simulink model "Farmakokinetika"  (R2022b)
settings: Solver=VariableStepAuto  StartTime=0.0  StopTime=600  RelTol=1e-3
values from neighbouring files (symbols this model uses):
  Gb = 153    [params.m]
  Ib = 6.5    [params.m]
  ki = Pop(i,3)    [fitness.m]    (also in gen3.m = best_ch(3,end); params.m = 0.1629)
  p2 = Pop(i,1)    [fitness_dk.m]    (also in params.m = best_ch(1,end))
  Sg = 0    [params.m]
  Si = Pop(i,2)    [fitness_dk.m]    (also in params.m = best_ch(2,end))
  Ti = Pop(i,1)    [fitness.m]    (also in gen3.m = best_ch(1,end); params.m = 45.383)
  v = 281.218    [fitness.m]    (also in fitness_dk.m; gen3.m = 281.28; params.m = 281.28)
  Vg = 1.467    [params.m]
  Vi = Pop(i,2)    [fitness.m]    (also in gen3.m = best_ch(2,end); params.m = 139.094)
  weight = 64.4    [params.m]
settings Model: Creator=DFUNDO  LastModifiedBy=DFUNDO

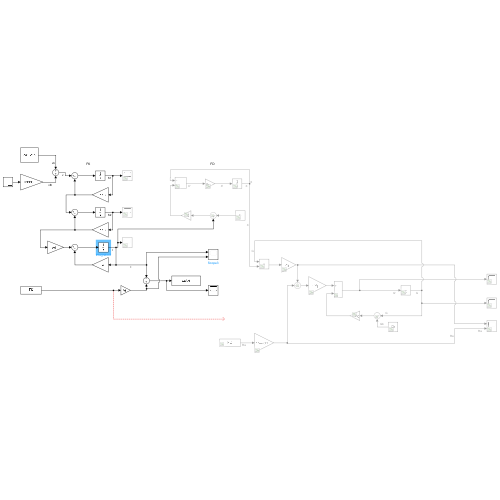
[thumbnail: Simulink's stored preview of the top-level diagram]
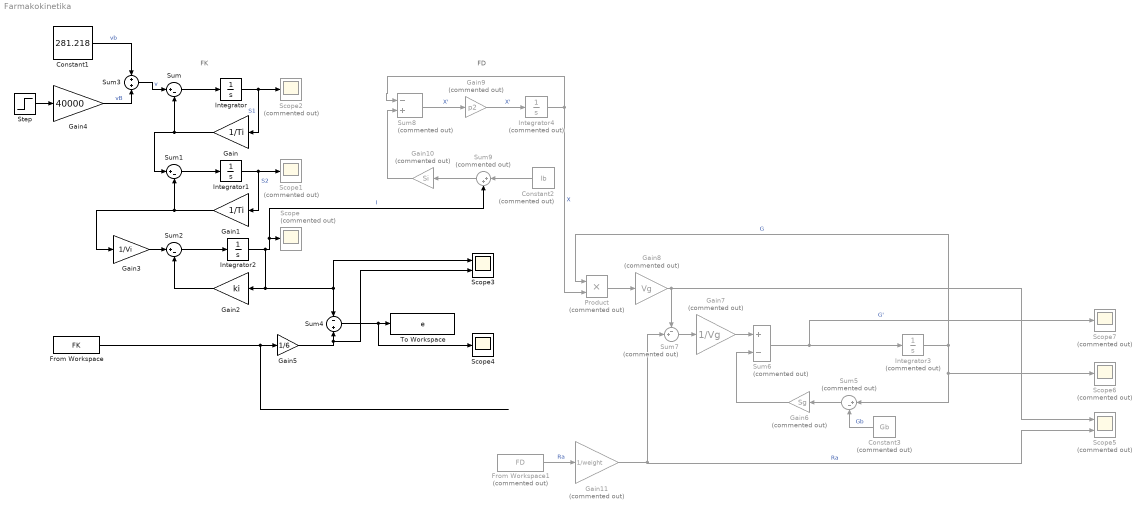
== system Farmakokinetika ==
  note: FD
  note: FK
  Constant1 : Constant  Value=281.218
  Constant2 : Constant  Commented=on  Value=Ib
  Constant3 : Constant  Commented=on  Value=Gb
  From Workspace : FromWorkspace  VariableName=FK
  From Workspace1 : FromWorkspace  Commented=on  VariableName=FD
  Gain : Gain  Gain=1/Ti
  Gain1 : Gain  Gain=1/Ti
  Gain10 : Gain  Commented=on  Gain=Si
  Gain11 : Gain  Commented=on  Gain=1/weight
  Gain2 : Gain  Gain=ki
  Gain3 : Gain  Gain=1/Vi
  Gain4 : Gain  Gain=40000
  Gain5 : Gain  Gain=1/6
  Gain6 : Gain  Commented=on  Gain=Sg
  Gain7 : Gain  Commented=on  Gain=1/Vg
  Gain8 : Gain  Commented=on  Gain=Vg
  Gain9 : Gain  Commented=on  Gain=p2
  Integrator : Integrator  InitialCondition=Ti*v
  Integrator1 : Integrator  InitialCondition=Ti*v
  Integrator2 : Integrator  InitialCondition=v/(Vi*ki)
  Integrator3 : Integrator  Commented=on  InitialCondition=Gb
  Integrator4 : Integrator  Commented=on
  Product : Product  Commented=on
  Scope{,1..2,6..7} (5 alike) : Scope  Commented=on
  Scope3 : Scope  NumInputPorts=2
  Scope4 : Scope
  Scope5 : Scope  Commented=on  NumInputPorts=2
  Step : Step  Time=5  Before=1  After=0  SampleTime=0
  Sum : Sum  Inputs=|+-
  Sum1 : Sum  Inputs=|+-
  Sum2 : Sum  Inputs=|+-
  Sum3 : Sum
  Sum4 : Sum  Inputs=-+
  Sum5 : Sum  Commented=on  Inputs=|+-
  Sum6 : Sum  Commented=on  Inputs=+-
  Sum7 : Sum  Commented=on  Inputs=-+|
  Sum8 : Sum  Commented=on  Inputs=-+
  Sum9 : Sum  Commented=on  Inputs=|++
  To Workspace : ToWorkspace  VariableName=e  SampleTime=-1
      settings: Save2DSignal=2-D array (concatenate along first dimension)
  wires:
  Integrator/1 -> Gain/1, Scope2/1  "S1"
  Gain/1 -> Sum/2, Sum1/1
  Sum/1 -> Integrator/1
  Sum3/1 -> Sum/1  "v"
  Integrator1/1 -> Scope1/1, Gain1/1  "S2"
  Gain1/1 -> Gain3/1, Sum1/2
  Sum1/1 -> Integrator1/1
  Sum2/1 -> Integrator2/1
  Gain2/1 -> Sum2/2
  Integrator2/1 -> Sum4/1, Scope3/1, Gain2/1, Sum9/2, Scope/1  "I"
  Gain3/1 -> Sum2/1
  Constant1/1 -> Sum3/1  "vb"
  Gain4/1 -> Sum3/2  "vB"
  Step/1 -> Gain4/1
  From Workspace/1 -> Gain5/1
  Sum4/1 -> Scope4/1, To Workspace/1
  Gain5/1 -> Scope3/2, Sum4/2
  Integrator3/1 -> Product/1, Sum5/1, Scope6/1  "G"
  Sum6/1 -> Scope7/1, Integrator3/1  "G'"
  Sum5/1 -> Gain6/1
  Constant3/1 -> Sum5/2  "Gb"
  Gain6/1 -> Sum6/2
  Product/1 -> Gain8/1
  Sum7/1 -> Gain7/1
  Gain8/1 -> Scope5/1, Sum7/1
  Gain7/1 -> Sum6/1
  Integrator4/1 -> Product/2, Sum8/1  "X"
  Gain9/1 -> Integrator4/1  "X'"
  Sum8/1 -> Gain9/1  "X'"
  Gain10/1 -> Sum8/2
  Constant2/1 -> Sum9/1
  Sum9/1 -> Gain10/1
  Gain11/1 -> Scope5/2, Sum7/2  "Ra"
  From Workspace1/1 -> Gain11/1  "Ra"
